simulink model "VVI_FINAL"  (R2020a)
settings: Solver=FixedStepAuto  StartTime=0.0  StopTime=10.0  FixedStep=1e-3  RelTol=1e-3  EnableMultiTasking=on
settings Model: ExtModeTrigDuration=5  Creator=emily  LastModifiedBy=emily
settings OptimizationCC: EnhancedBackFolding=on  PassReuseOutputArgsAs=Individual arguments  ZeroExternalMemoryAtStartup=off  ZeroInternalMemoryAtStartup=off  MaxStackSize=64  OptimizeBlockOrder=speed  DifferentSizesBufferReuse=on  OptimizationCustomize=off  EfficientTunableParamExpr=on
settings DebuggingCC: ParameterTunabilityLossMsg=error
settings HardwareCC: ProdBitPerPointer=32  ProdBitPerSizeT=32  ProdBitPerPtrDiffT=32  ProdLargestAtomicInteger=Long  ProdLargestAtomicFloat=Double  ProdWordSize=32  ProdHWDeviceType=ARM Compatible->ARM Cortex
settings SFSimCC: MATLABDynamicMemAlloc=off
settings RTWCC: SystemTargetFile=ert.tlc  HardwareBoard=NXP FRDM-K64F  TemplateMakefile=ert_default_tmf  Toolchain=GNU Tools for ARM Embedded Processors
settings CodeAppCC: ForceParamTrailComments=on  IgnoreCustomStorageClasses=off  OperatorAnnotations=on  SimulinkDataObjDesc=on  SFDataObjDesc=on  InsertBlockDesc=on

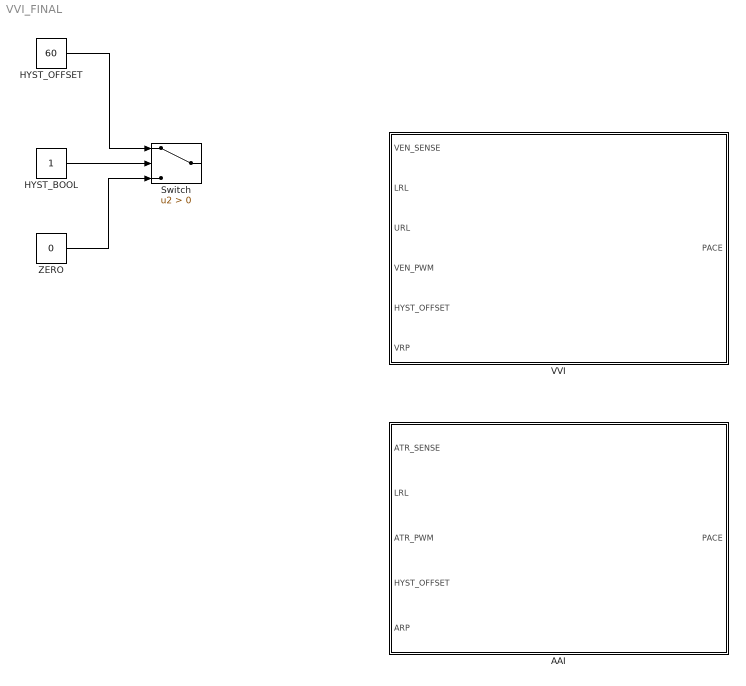
== system VVI_FINAL ==
  AAI : Stateflow chart  TreatAsAtomicUnit=on
  HYST_BOOL : Constant
  HYST_OFFSET : Constant  Value=60  OutDataTypeStr=double
  Switch : Switch  Criteria=u2 > Threshold
  VVI : Stateflow chart  TreatAsAtomicUnit=on
  ZERO : Constant  Value=0
  wires:
  HYST_OFFSET/1 -> Switch/1
  HYST_BOOL/1 -> Switch/2
  ZERO/1 -> Switch/3

== stateflow chart VVI_FINAL/AAI ==
  state WAIT
    entry:
    PACE = 0;
  state PACE
    entry:
    PACE = 1;
  state REFRACTORY
    entry:
    PACE = 0;
  (default) -> WAIT
  WAIT -> WAIT [order 2] : [ATR_SENSE == 1]
  WAIT -> PACE [order 1] : after(60000/LRL+HYST_OFFSET,msec)
  REFRACTORY -> WAIT : after(ARP, msec)
  PACE -> REFRACTORY : after(ATR_PWM,msec)
  data: ATR_SENSE input boolean; LRL input; ATR_PWM input; HYST_OFFSET input; PACE output; ARP input

== stateflow chart VVI_FINAL/VVI ==
  state WAIT
    entry:
    PACE = 0;
  state PACE
    entry:
    PACE = 1;
  state REFRACTORY
    entry:
    PACE = 0;
  (default) -> WAIT
  WAIT -> WAIT [order 2] : [VEN_SENSE == 1]
  WAIT -> PACE [order 1] : after(60000/LRL+HYST_OFFSET,msec)
  REFRACTORY -> WAIT : after(VRP, msec)
  PACE -> REFRACTORY : after(VEN_PWM,msec)
  data: VEN_SENSE input boolean; LRL input; URL input; VEN_PWM input; HYST_OFFSET input; PACE output; VRP input
